simulink library "pv_celltemp_sapm"  (R2018b)
settings: Solver=VariableStepAuto  StartTime=0.0  StopTime=10.0  RelTol=1e-3
settings Model: Creator=P41573  LastModifiedBy=P41573
settings SFSimCC: SimUseLocalCustomCode=off
settings RTWCC: RTWUseLocalCustomCode=off
settings CodeAppCC: StateflowObjectComments=on

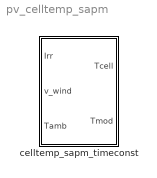
== system pv_celltemp_sapm ==
  celltemp_sapm_timeconst : Subsystem  mask{E0=1000, a=-3.56, b=-0.075, dTc=2, TypeMount=Glass/cell/glass - Open rack, tini=25}
      mask prompts: E0 "Reference Irradiation for deltaT (W/m2)"; a "SAPM Parameter - a [-]"; b "SAPM Parameter - b [s/m]"; dTc "SAPM Parameter - deltaT [K]"; TypeMount "Panel type / Mounting Option"; tini "initial cell temperature - [°C]"
      mask TypeOptions E0: pv_sapmcelltemp/E0
      mask TypeOptions a: pv_sapmcelltemp/a_wind
      mask TypeOptions b: pv_sapmcelltemp/b_wind
      mask TypeOptions dTc: pv_sapmcelltemp/deltaT
      mask TypeOptions TypeMount: <propagated> | <user defined> | Glass/cell/glass - Open rack | Glass/cell/glass - Close roof mount | Glass/cell/polymer sheet - Open rack | Glass/cell/polymer sheet - Insulated back | Polymer/thin-film/steel - Open rack
      mask Callback TypeMount: [ok, param] = CarnotCallbacks_PvCelltempSapm(gcbh);

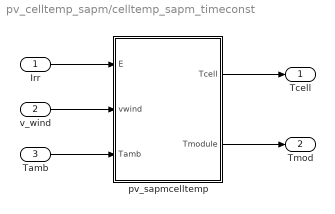
== system pv_celltemp_sapm/celltemp_sapm_timeconst ==
  Irr : Inport
  v_wind : Inport  Port=2
  Tamb : Inport  Port=3
  pv_sapmcelltemp : MATLAB Function  TreatAsAtomicUnit=on  mask{E0=E0, a_wind=a, b_wind=b, deltaT=dTc}
      mask prompts: E0 "Reference Irradiation for deltaT (W/m2)"; a_wind "SAPM Parameter - a [-]"; b_wind "SAPM Parameter - b [s/m]"; deltaT "SAPM Parameter - deltaT [K]"
  Tcell : Outport
  Tmod : Outport  Port=2
  wires:
  Irr/1 -> pv_sapmcelltemp/1(E)
  v_wind/1 -> pv_sapmcelltemp/2(vwind)
  Tamb/1 -> pv_sapmcelltemp/3(Tamb)
  pv_sapmcelltemp/1(Tcell) -> Tcell/1
  pv_sapmcelltemp/2(Tmodule) -> Tmod/1

== matlab function pv_celltemp_sapm/celltemp_sapm_timeconst/pv_sapmcelltemp ==
  data: E input; vwind input; Tamb input; Tcell output; Tmodule output; E0 parameter; a_wind parameter; b_wind parameter; deltaT parameter
function [Tcell,Tmodule] = pv_sapmcelltemp(E, vwind, Tamb, E0, a_wind, b_wind, deltaT)

%% PVL_SAPMCELLTEMP Estimate cell temperature from irradiance, windspeed, ambient temperature, and module parameters (SAPM)
% Syntax
%   Tcell = pvl_sapmcelltemp(E, E0, a, b, windspeed, Tamb, deltaT)
%   [Tcell Tmodule] = pv_sapmcelltemp(E, E0, a, b, windspeed, Tamb, deltaT)
%
% Description
%   Estimate cell and module temperatures per the Sandia PV Array
%   Performance model (SAPM, SAND2004-3535), when given the incident
%   irradiance, wind speed, ambient temperature, and SAPM module
%   parameters.
%
% Inputs
%   E - Total incident irradiance in W/m^2. E must be a scalar or a vector
%     of the same size as windspeed, and Tamb. Must be >=0.
%   E0 - Reference irradiance used when determining delta T, in W/m^2. E0
%     must be a scalar. Must be >=0;
%   a - SAPM module parameter for establishing the upper limit for module 
%     temperature at low wind speeds and high solar irradiance (see SAPM
%     eqn. 11). Must be a scalar.
%   b - SAPM module parameter for establishing the rate at which the module
%     temperature drops as wind speed increases (see SAPM eqn. 11). Must be
%     a scalar.
%   windspeed - Wind speed in m/s at a height of 10 meters. windspeed must
%     be a scalar or a vector of the same size as E and Tamb. Must be >=0;
%   Tamb - Ambient dry bulb temperature in degrees C. Tamb must be a scalar
%     or a vector of the same size as windspeed and E. Must be >= -273.15.
%   deltaT - SAPM module parameter giving the temperature difference
%     between the cell and module back surface at the reference irradiance,
%     E0. Must be a numeric scalar >=0.
%  
% References
%   [1] King, D. et al, 2004, "Sandia Photovoltaic Array Performance Model", SAND Report
%   3535, Sandia National Laboratories, Albuquerque, NM
%
%%
Tmodule = E.*(exp(a_wind+b_wind.*vwind))+Tamb;
Tcell = Tmodule + E./E0.*deltaT;
